simulink model "SimObserverExample"  (Simulink 7.8)
settings: Solver=ode45  StartTime=0.0  StopTime=20.0  RelTol=1e-3
settings Model: Creator=amiria  LastModifiedBy=rafieem
settings DataIOCC: SignalLoggingSaveFormat=Dataset
settings GRTTargetCC: CombineOutputUpdateFcns=on

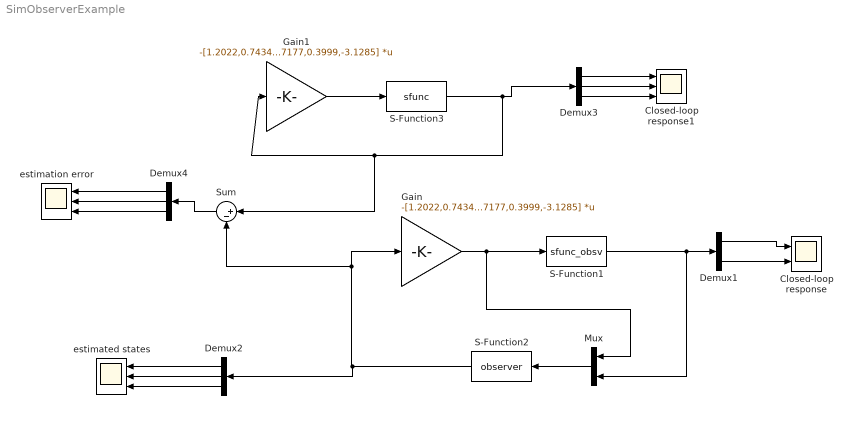
== system SimObserverExample ==
  Closed-loop response : Scope  NumInputPorts=2
      settings: YMin=-5~-5  YMax=5~5
  Closed-loop response1 : Scope  NumInputPorts=3
      settings: YMin=-5~-5~-5  YMax=5~5~5  SaveName=ScopeData2
  Demux1 : Demux  Outputs=2
  Demux2 : Demux  Outputs=3
  Demux3 : Demux  Outputs=3
  Demux4 : Demux  Outputs=3
  Gain : Gain  Gain=-[1.2022,0.7434,-5.6941;0.7177,0.3999,-3.1285]  Multiplication=Matrix(K*u)
  Gain1 : Gain  Gain=-[1.2022,0.7434,-5.6941;0.7177,0.3999,-3.1285]  Multiplication=Matrix(K*u)
  Mux : Mux  Inputs=2
  S-Function1 : S-Function  FunctionName=sfunc_obsv  EnableBusSupport=off
  S-Function2 : S-Function  FunctionName=observer  EnableBusSupport=off
  S-Function3 : S-Function  FunctionName=sfunc  EnableBusSupport=off
  Sum : Sum  Inputs=|+-
  estimated states : Scope  NumInputPorts=3
      settings: YMin=-5~-5~-5  YMax=5~5~5
  estimation error : Scope  NumInputPorts=3
      settings: YMin=-5~-5~-5  YMax=5~5~5  SaveName=ScopeData3
  wires:
  Gain/1 -> Mux/1, S-Function1/1
  Demux1/1 -> Closed-loop response/1
  Demux1/2 -> Closed-loop response/2
  S-Function1/1 -> Demux1/1, Mux/2
  S-Function2/1 -> Demux2/1, Sum/2, Gain/1
  Mux/1 -> S-Function2/1
  Demux2/1 -> estimated states/1
  Demux2/2 -> estimated states/2
  Demux2/3 -> estimated states/3
  Gain1/1 -> S-Function3/1
  Demux3/1 -> Closed-loop response1/1
  Demux3/2 -> Closed-loop response1/2
  S-Function3/1 -> Sum/1, Gain1/1, Demux3/1
  Demux3/3 -> Closed-loop response1/3
  Demux4/1 -> estimation error/1
  Demux4/2 -> estimation error/2
  Demux4/3 -> estimation error/3
  Sum/1 -> Demux4/1
